simulink library "nmc"  (R2015b)
settings: Solver=ode45  SolverMode=SingleTasking  StartTime=0.0  StopTime=10.0  RelTol=1e-3
undefined symbols (not defined in the file): AFOFS_DIM, alphaFmGas, alphaFmGlu, alphaFmHam, alphaFmSol, alphaFmVas, alphaLceHam, alphaLceHfl, alphaLceTa, alphaLceTa1, Amp, amp_var, c, c_jointstop, CPG, D1G_HAT, DeltaThRef, eref, FmaxGAS, FmaxGLU, FmaxHAM, FmaxHFL, FmaxSOL, FmaxTA, FmaxVAS, freq, freq_var, GainDeltaTheta, GainGAS, GainGLU, GainHAM, GainHAMHFL, GainHFL, GainKneOverExt, GainSOL, GainSOLTA, GainTA, GainVAS, K, K_swing, KneePh23Offset, LceOffsetHAM, LceOffsetHFL, LceOffsetTA, left, LongDelay, loptGAS, loptGLU, loptHAM, loptHFL, loptSOL, loptTA, loptVAS, Lphi230, lslackGAS, lslackGLU, lslackHAM, lslackHFL, lslackSOL, lslackTA ... (+66)
libraries: nmc x94, simulink x29, simulink_extras x17
(part 3 of 5)

== system nmc/NMC Muscles/HFL&HAM Muscles/HFL&HAM Control ==
  note: HFL with HAM Control
  LceHFL : Inport
  LceHam : Inport  Port=2
  FmHam : Inport  Port=3
  Theta : Inport  Port=4
  dTheta : Inport  Port=5
  CLdxThigh : Inport  Port=6
  OLonCL : Inport  Port=7
  StanceSwing : Inport  Port=8
  "ANMC STIM " : Concatenate  NumInputs=1
  ANMC STIM 1 : Concatenate  NumInputs=1
  Demux : Demux  Outputs=2
  Logical Operator : Logic  Operator=NOT  AllPortsSameDT=off  OutDataTypeStr=boolean
  Mux1 : Mux  Inputs=2
  Mux2 : Mux  Inputs=2
  Saturation17 : Saturate  UpperLimit=1  LowerLimit=0.01  ZeroCross=off
  Stance Phase : Subsystem  TreatAsAtomicUnit=on
  Sum18 : Sum
  Swing Phase : Subsystem  TreatAsAtomicUnit=on
  StimHFL : Outport
  StimHAM : Outport  Port=2
  wires:
  ANMC STIM 1/1 -> StimHAM/1
  "ANMC STIM "/1 -> StimHFL/1
  Demux/1 -> "ANMC STIM "/1
  Demux/2 -> ANMC STIM 1/1
  OLonCL/1 -> Stance Phase/4(OLonCL)
  Swing Phase/2(StimHAM) -> Mux1/2
  Mux1/1 -> Sum18/2
  Mux2/1 -> Sum18/1
  Saturation17/1 -> Demux/1
  Sum18/1 -> Saturation17/1
  StanceSwing/1 -> Logical Operator/1, Stance Phase/Enable
  LceHFL/1 -> Swing Phase/2(LceHFL)
  Stance Phase/2(StimHAM) -> Mux2/2
  Stance Phase/1(StimHFL) -> Mux2/1
  CLdxThigh/1 -> Stance Phase/3(CLdxThigh [N])
  Stance Phase/3(Delta_Theta) -> Swing Phase/1(Delta_Theta)
  FmHam/1 -> Swing Phase/4(FmHAM)
  LceHam/1 -> Swing Phase/3(LceHAM)
  Swing Phase/1(StimHFL) -> Mux1/1
  dTheta/1 -> Stance Phase/2(dTheta [rad/s])
  Theta/1 -> Stance Phase/1(Theta)
  Logical Operator/1 -> Swing Phase/Enable

== system nmc/NMC Muscles/SOL&TA Muscles/SOL Actuation ==
  note: SOL Actuation
  phiAnkle : Inport
  StimSOL : Inport  Port=2
  " SOL" : Subsystem
  " SOL Golgi Tendon Organs" : Gain
  Mux3 : Mux  Inputs=5
  Product : Product  RndMeth=Zero
  SOL Link : Subsystem
  SOL loop delay : TransportDelay  DelayTime=LongDelay
  Terminator3 : Terminator
  TauSOL : Outport
  FmSOL : Outport  Port=2
  tag scope: SOLL_VM=global
  wires:
  SOL loop delay/1 -> FmSOL/1
  " SOL Golgi Tendon Organs"/1 -> SOL loop delay/1
  StimSOL/1 -> " SOL"/1(STIM)
  phiAnkle/1 -> SOL Link/1(phi12 [rad])
  " SOL"/4(Lse) -> Mux3/4
  " SOL"/3(Vce) -> Mux3/3
  " SOL"/2(Lce) -> Mux3/2
  Mux3/1 -> Terminator3/1, [SOLL_VM]
  " SOL"/5(A) -> Mux3/5
  Product/1 -> TauSOL/1
  SOL Link/2(lever [m]) -> Product/1
  SOL Link/1(lmtc [m]) -> " SOL"/2(lmtc [m])
  " SOL"/1(Fmtc) -> Mux3/1, " SOL Golgi Tendon Organs"/1, Product/2

== system nmc/NMC Muscles/SOL&TA Muscles/SOL&TA Control ==
  note: SOL with TA Control
  LceTA : Inport
  FmSOL : Inport  Port=2
  StanceSwing : Inport  Port=3
  " Stance Phase" : Subsystem  TreatAsAtomicUnit=on
  "ANMC STIM " : Concatenate  NumInputs=1
  ANMC STIM 1 : Concatenate  NumInputs=1
  Demux : Demux  Outputs=2
  Logical Operator : Logic  Operator=NOT  AllPortsSameDT=off  OutDataTypeStr=boolean
  Mux1 : Mux  Inputs=2
  Mux2 : Mux  Inputs=2
  Saturation17 : Saturate  UpperLimit=1  LowerLimit=0.01  ZeroCross=off
  Sum18 : Sum
  Swing Phase : Subsystem  TreatAsAtomicUnit=on
  StimTA : Outport
  StimSOL : Outport  Port=2
  wires:
  ANMC STIM 1/1 -> StimSOL/1
  "ANMC STIM "/1 -> StimTA/1
  Demux/1 -> "ANMC STIM "/1
  Demux/2 -> ANMC STIM 1/1
  Swing Phase/2(StimSOL) -> Mux1/2
  Mux1/1 -> Sum18/2
  Mux2/1 -> Sum18/1
  Saturation17/1 -> Demux/1
  Sum18/1 -> Saturation17/1
  " Stance Phase"/2(StimSOL) -> Mux2/2
  " Stance Phase"/1(StimTA) -> Mux2/1
  Swing Phase/1(StimTA) -> Mux1/1
  LceTA/1 -> " Stance Phase"/2(LceTA), Swing Phase/1(LceTA)
  StanceSwing/1 -> Logical Operator/1, " Stance Phase"/Enable
  FmSOL/1 -> " Stance Phase"/1(FmSOL)
  Logical Operator/1 -> Swing Phase/Enable

== system nmc/NMC Muscles/SOL&TA Muscles/TA Actuation ==
  note: TA Actuation
  phiAnkle : Inport
  StimTA : Inport  Port=2
  " TA Muscle Spindles" : Gain  Gain=1/loptTA
  " TA loop delay" : TransportDelay  DelayTime=LongDelay
  Gain : Gain  Gain=-1
  Mux8 : Mux  Inputs=5
  Product1 : Product  RndMeth=Zero
  Saturation2 : Saturate  UpperLimit=inf  LowerLimit=0  ZeroCross=off
  Stimulation Bias3 : Constant  Value=LceOffsetTA
  Sum21 : Sum  Inputs=-+|  SaturateOnIntegerOverflow=on  InputSameDT=on  OutDataTypeStr=Inherit: Same as first input
  TA : Subsystem
  TA Link : Subsystem
  Terminator8 : Terminator
  LceTA : Outport
  TauTa : Outport  Port=2
  tag scope: TAL_VM=global
  wires:
  Gain/1 -> TauTa/1
  " TA loop delay"/1 -> LceTA/1
  StimTA/1 -> TA/1(STIM)
  Product1/1 -> Gain/1
  Saturation2/1 -> " TA loop delay"/1
  Stimulation Bias3/1 -> Sum21/1
  phiAnkle/1 -> TA Link/1(phi12 [rad])
  TA/3(Vce) -> Mux8/3
  TA/4(Lse) -> Mux8/4
  Mux8/1 -> Terminator8/1, [TAL_VM]
  Sum21/1 -> Saturation2/1
  " TA Muscle Spindles"/1 -> Sum21/2
  TA Link/2(lever [m]) -> Product1/2
  TA Link/1(lmtc [m]) -> TA/2(lmtc [m])
  TA/5(A) -> Mux8/5
  TA/2(Lce) -> Mux8/2, " TA Muscle Spindles"/1
  TA/1(Fmtc) -> Mux8/1, Product1/1

== system nmc/NMC Muscles/VAS Muscle/VAS Actuation  ==
  note: VAS Actuation
  phiKnee : Inport
  StimVas : Inport  Port=2
  " VAS Golgi Tendon Organs" : Gain
  Gain : Gain  Gain=-1
  Mux9 : Mux  Inputs=5
  Product4 : Product  RndMeth=Zero
  Terminator9 : Terminator
  VAS : Subsystem
  VAS Link : Subsystem
  VAS loop delay : TransportDelay  DelayTime=MidDelay
  TauVas : Outport
  FmVas : Outport  Port=2
  tag scope: VASR_VM=global
  wires:
  VAS loop delay/1 -> FmVas/1
  " VAS Golgi Tendon Organs"/1 -> VAS loop delay/1
  Gain/1 -> TauVas/1
  StimVas/1 -> VAS/1(STIM)
  phiKnee/1 -> VAS Link/1(phi23 [rad])
  VAS/2(Lce) -> Mux9/2
  VAS/3(Vce) -> Mux9/3
  VAS/4(Lse) -> Mux9/4
  Mux9/1 -> Terminator9/1, [VASR_VM]
  VAS Link/2(lever [m]) -> Product4/1
  VAS/1(Fmtc) -> Mux9/1, " VAS Golgi Tendon Organs"/1, Product4/2
  VAS/5(A) -> Mux9/5
  Product4/1 -> Gain/1
  VAS Link/1(lmtu [m]) -> VAS/2(lmtc [m])

== system nmc/NMC Muscles/VAS Muscle/VAS Control ==
  note: VAS Control
  FmVAS : Inport
  OLdxThigh : Inport  Port=2
  OLonCL : Inport  Port=3
  CLKneeState : Inport  Port=4
  StanceSwing : Inport  Port=5
  " Swing Phase" : Subsystem  TreatAsAtomicUnit=on
  "ANMC STIM " : Concatenate  NumInputs=1
  Logical Operator : Logic  Operator=NOT  AllPortsSameDT=off  OutDataTypeStr=boolean
  Saturation17 : Saturate  UpperLimit=1  LowerLimit=0.01  ZeroCross=off
  Stance Phase : Subsystem  TreatAsAtomicUnit=on
  Sum18 : Sum
  StimVAS : Outport
  wires:
  "ANMC STIM "/1 -> StimVAS/1
  CLKneeState/1 -> Stance Phase/1(CLKneeState)
  OLonCL/1 -> Stance Phase/2(OLonCL)
  OLdxThigh/1 -> Stance Phase/3(OLdxThigh [N])
  Stance Phase/1(StimVAS) -> Sum18/1
  Saturation17/1 -> "ANMC STIM "/1
  Sum18/1 -> Saturation17/1
  " Swing Phase"/1(StimVAS) -> Sum18/2
  StanceSwing/1 -> Stance Phase/Enable, Logical Operator/1
  FmVAS/1 -> Stance Phase/4(FmVAS)
  Logical Operator/1 -> " Swing Phase"/Enable

== system nmc/NMC Sensors/FootSensor/Cross Influence Detection ==
  note: left leg is leading
  note: right leg is leading
  note: Double Support Cross Influences
  LStance : Inport  OutDataTypeStr=double
  RStance : Inport  Port=2  OutDataTypeStr=double
  DSup ends : HitCross  HitCrossingOffset=0.5  HitCrossingDirection=falling  ZeroCross=off
  Double Support? : Logic  AllPortsSameDT=off
  Double Support?1 : Logic  AllPortsSameDT=off
  Double Support?4 : Logic  AllPortsSameDT=off
  Flight? : Logic  Operator=NOR  AllPortsSameDT=off
  LLeg starts DSup : HitCross  HitCrossingOffset=0.5  HitCrossingDirection=rising  ZeroCross=off
  Memory : Memory
  Memory3 : Memory
  RLeg starts DSup : HitCross  HitCrossingOffset=0.5  HitCrossingDirection=rising  ZeroCross=off
  S-R Flip-Flop : simulink_extras/Flip Flops/S-R Flip-Flop  initial_condition=0
  S-R Flip-Flop1 : simulink_extras/Flip Flops/S-R Flip-Flop  initial_condition=0
  Terminator1 : Terminator
  Terminator2 : Terminator
  RonL : Outport  OutDataTypeStr=double
  Flight : Outport  Port=2  OutDataTypeStr=double
  LonR : Outport  Port=3  OutDataTypeStr=double
  wires:
  S-R Flip-Flop1/1 -> RonL/1
  Flight?/1 -> Flight/1
  S-R Flip-Flop/1 -> LonR/1
  Double Support?/1 -> Double Support?4/2, Double Support?1/1, DSup ends/1
  RStance/1 -> Flight?/2, Double Support?/2, Memory/1
  Memory3/1 -> LLeg starts DSup/1
  Double Support?4/1 -> S-R Flip-Flop/1
  LLeg starts DSup/1 -> Double Support?4/1
  LStance/1 -> Flight?/1, Double Support?/1, Memory3/1
  Memory/1 -> RLeg starts DSup/1
  S-R Flip-Flop1/2 -> Terminator2/1
  DSup ends/1 -> S-R Flip-Flop1/2, S-R Flip-Flop/2
  S-R Flip-Flop/2 -> Terminator1/1
  RLeg starts DSup/1 -> Double Support?1/2
  Double Support?1/1 -> S-R Flip-Flop1/1

== system nmc/NMC Sensors/FootSensor/Cross Influence Detection1 ==
  note: Double Support Cross Influences
  note: right leg is leading
  note: left leg is leading
  LStance : Inport  OutDataTypeStr=double
  RStance : Inport  Port=2  OutDataTypeStr=double
  Data Type Conversion{1..4} (4 alike) : DataTypeConversion
  Detect Decrease : simulink/Logic and Bit Operations/Detect Decrease  vinit=1.0  InputProcessing=Inherited  OutDataTypeStr=boolean
  Detect Increase : simulink/Logic and Bit Operations/Detect Increase  vinit=0.0  InputProcessing=Inherited  OutDataTypeStr=boolean
  Detect Increase1 : simulink/Logic and Bit Operations/Detect Increase  vinit=0.0  InputProcessing=Inherited  OutDataTypeStr=boolean
  Double Support? : Logic  AllPortsSameDT=off
  Double Support?1 : Logic  AllPortsSameDT=off
  Double Support?4 : Logic  AllPortsSameDT=off
  Flight? : Logic  Operator=NOR  AllPortsSameDT=off
  Memory : Memory
  Memory3 : Memory
  S-R Flip-Flop : simulink_extras/Flip Flops/S-R Flip-Flop  initial_condition=0
  S-R Flip-Flop1 : simulink_extras/Flip Flops/S-R Flip-Flop  initial_condition=0
  Terminator1 : Terminator
  Terminator2 : Terminator
  RonL : Outport  OutDataTypeStr=double
  Flight : Outport  Port=2  OutDataTypeStr=double
  LonR : Outport  Port=3  OutDataTypeStr=double
  wires:
  Double Support?1/1 -> S-R Flip-Flop1/1
  Detect Increase/1 -> Double Support?1/2
  S-R Flip-Flop/2 -> Terminator1/1
  S-R Flip-Flop1/2 -> Terminator2/1
  Memory/1 -> Detect Increase/1
  LStance/1 -> Memory3/1, Double Support?/1, Flight?/1
  Detect Increase1/1 -> Double Support?4/1
  Double Support?4/1 -> S-R Flip-Flop/1
  Memory3/1 -> Detect Increase1/1
  RStance/1 -> Memory/1, Double Support?/2, Flight?/2
  Double Support?/1 -> Data Type Conversion4/1, Double Support?1/1, Double Support?4/2
  S-R Flip-Flop/1 -> Data Type Conversion2/1
  Flight?/1 -> Data Type Conversion1/1
  S-R Flip-Flop1/1 -> Data Type Conversion3/1
  Data Type Conversion1/1 -> Flight/1
  Data Type Conversion2/1 -> LonR/1
  Data Type Conversion3/1 -> RonL/1
  Detect Decrease/1 -> S-R Flip-Flop/2, S-R Flip-Flop1/2
  Data Type Conversion4/1 -> Detect Decrease/1

== system nmc/Parameter variation/Alpha variation/Alpha Variation ==
  alpha : EnablePort  ShowOutputPort=on
  Gain : Gain  Gain=10
  Gain1 : Gain  Gain=0.1
  Ramp : simulink/Sources/Ramp  slope=0.05  start=2  X0=0
  Rounding Function : Rounding  Operator=round
  Saturation : Saturate  UpperLimit=1  LowerLimit=0
  Switch : Switch  Threshold=1
  "alphaOut " : Outport
  wires:
  Switch/1 -> "alphaOut "/1
  Ramp/1 -> Gain/1
  alpha/1 -> Switch/2, Switch/3
  Saturation/1 -> Switch/1
  Gain/1 -> Rounding Function/1
  Rounding Function/1 -> Gain1/1
  Gain1/1 -> Saturation/1

== system nmc/Parameter variation/Alpha variation/Alpha Variation1 ==
  alpha : EnablePort  ShowOutputPort=on
  Gain : Gain  Gain=10
  Gain1 : Gain  Gain=0.1
  Ramp : simulink/Sources/Ramp  slope=0.05  start=2  X0=0
  Rounding Function : Rounding  Operator=round
  Saturation : Saturate  UpperLimit=1  LowerLimit=0
  Switch : Switch  Threshold=1
  "alphaOut " : Outport
  wires:
  Switch/1 -> "alphaOut "/1
  Ramp/1 -> Gain/1
  alpha/1 -> Switch/2, Switch/3
  Saturation/1 -> Switch/1
  Gain/1 -> Rounding Function/1
  Rounding Function/1 -> Gain1/1
  Gain1/1 -> Saturation/1

== system nmc/Parameter variation/Alpha variation/Alpha Variation2 ==
  alpha : EnablePort  ShowOutputPort=on
  Gain : Gain  Gain=10
  Gain1 : Gain  Gain=0.1
  Ramp : simulink/Sources/Ramp  slope=0.05  start=2  X0=0
  Rounding Function : Rounding  Operator=round
  Saturation : Saturate  UpperLimit=1  LowerLimit=0
  Switch : Switch  Threshold=1
  "alphaOut " : Outport
  wires:
  Switch/1 -> "alphaOut "/1
  Ramp/1 -> Gain/1
  alpha/1 -> Switch/2, Switch/3
  Saturation/1 -> Switch/1
  Gain/1 -> Rounding Function/1
  Rounding Function/1 -> Gain1/1
  Gain1/1 -> Saturation/1

== system nmc/Parameter variation/Alpha variation/Alpha Variation3 ==
  alpha : EnablePort  ShowOutputPort=on
  Gain : Gain  Gain=10
  Gain1 : Gain  Gain=0.1
  Ramp : simulink/Sources/Ramp  slope=0.05  start=2  X0=0
  Rounding Function : Rounding  Operator=round
  Saturation : Saturate  UpperLimit=1  LowerLimit=0
  Switch : Switch  Threshold=1
  "alphaOut " : Outport
  wires:
  Switch/1 -> "alphaOut "/1
  Ramp/1 -> Gain/1
  alpha/1 -> Switch/2, Switch/3
  Saturation/1 -> Switch/1
  Gain/1 -> Rounding Function/1
  Rounding Function/1 -> Gain1/1
  Gain1/1 -> Saturation/1

== system nmc/Parameter variation/Alpha variation/Alpha Variation4 ==
  alpha : EnablePort  ShowOutputPort=on
  Gain : Gain  Gain=10
  Gain1 : Gain  Gain=0.1
  Ramp : simulink/Sources/Ramp  slope=0.05  start=2  X0=0
  Rounding Function : Rounding  Operator=round
  Saturation : Saturate  UpperLimit=1  LowerLimit=0
  Switch : Switch  Threshold=1
  "alphaOut " : Outport
  wires:
  Switch/1 -> "alphaOut "/1
  Ramp/1 -> Gain/1
  alpha/1 -> Switch/2, Switch/3
  Saturation/1 -> Switch/1
  Gain/1 -> Rounding Function/1
  Rounding Function/1 -> Gain1/1
  Gain1/1 -> Saturation/1

== system nmc/Parameter variation/Alpha variation/Alpha Variation5 ==
  alpha : EnablePort  ShowOutputPort=on
  Gain : Gain  Gain=10
  Gain1 : Gain  Gain=0.1
  Ramp : simulink/Sources/Ramp  slope=0.05  start=2  X0=0
  Rounding Function : Rounding  Operator=round
  Saturation : Saturate  UpperLimit=1  LowerLimit=0
  Switch : Switch  Threshold=1
  "alphaOut " : Outport
  wires:
  Switch/1 -> "alphaOut "/1
  Ramp/1 -> Gain/1
  alpha/1 -> Switch/2, Switch/3
  Saturation/1 -> Switch/1
  Gain/1 -> Rounding Function/1
  Rounding Function/1 -> Gain1/1
  Gain1/1 -> Saturation/1

== system nmc/Parameter variation/Alpha variation/Alpha Variation6 ==
  alpha : EnablePort  ShowOutputPort=on
  Gain : Gain  Gain=10
  Gain1 : Gain  Gain=0.1
  Ramp : simulink/Sources/Ramp  slope=0.05  start=2  X0=0
  Rounding Function : Rounding  Operator=round
  Saturation : Saturate  UpperLimit=1  LowerLimit=0
  Switch : Switch  Threshold=1
  "alphaOut " : Outport
  wires:
  Switch/1 -> "alphaOut "/1
  Ramp/1 -> Gain/1
  alpha/1 -> Switch/2, Switch/3
  Saturation/1 -> Switch/1
  Gain/1 -> Rounding Function/1
  Rounding Function/1 -> Gain1/1
  Gain1/1 -> Saturation/1

== system nmc/Parameter variation/Alpha variation/Alpha Variation7 ==
  alpha : EnablePort  ShowOutputPort=on
  Gain : Gain  Gain=10
  Gain1 : Gain  Gain=0.1
  Ramp : simulink/Sources/Ramp  slope=0.05  start=2  X0=0
  Rounding Function : Rounding  Operator=round
  Saturation : Saturate  UpperLimit=1  LowerLimit=0
  Switch : Switch  Threshold=1
  "alphaOut " : Outport
  wires:
  Switch/1 -> "alphaOut "/1
  Ramp/1 -> Gain/1
  alpha/1 -> Switch/2, Switch/3
  Saturation/1 -> Switch/1
  Gain/1 -> Rounding Function/1
  Rounding Function/1 -> Gain1/1
  Gain1/1 -> Saturation/1

== system nmc/Parameter variation/Alpha variation/Alpha Variation8 ==
  alpha : EnablePort  ShowOutputPort=on
  Gain : Gain  Gain=10
  Gain1 : Gain  Gain=0.1
  Ramp : simulink/Sources/Ramp  slope=0.05  start=2  X0=0
  Rounding Function : Rounding  Operator=round
  Saturation : Saturate  UpperLimit=1  LowerLimit=0
  Switch : Switch  Threshold=1
  "alphaOut " : Outport
  wires:
  Switch/1 -> "alphaOut "/1
  Ramp/1 -> Gain/1
  alpha/1 -> Switch/2, Switch/3
  Saturation/1 -> Switch/1
  Gain/1 -> Rounding Function/1
  Rounding Function/1 -> Gain1/1
  Gain1/1 -> Saturation/1

== system nmc/Parameter variation/Amplitude Variation/Down ==
  Amp : Inport
  Enable : EnablePort
  Gain : Gain  Gain=10
  Gain1 : Gain  Gain=0.1
  Ramp : simulink/Sources/Ramp  slope=0.04  start=2  X0=0
  Rounding Function : Rounding  Operator=round
  Saturation : Saturate  UpperLimit=1.5  LowerLimit=0
  Subtract : Sum  Inputs=+-
  "AmpDown " : Outport
  wires:
  Saturation/1 -> Subtract/2
  Ramp/1 -> Gain/1
  Amp/1 -> Subtract/1
  Gain/1 -> Rounding Function/1
  Rounding Function/1 -> Gain1/1
  Gain1/1 -> Saturation/1
  Subtract/1 -> "AmpDown "/1

== system nmc/Parameter variation/Amplitude Variation/Off  ==
  Amp : Inport
  Enable : EnablePort
  "Amp " : Outport
  wires:
  Amp/1 -> "Amp "/1

== system nmc/Parameter variation/Amplitude Variation/Up ==
  Amp : Inport
  Enable : EnablePort
  Gain : Gain  Gain=10
  Gain1 : Gain  Gain=0.1
  Ramp : simulink/Sources/Ramp  slope=0.04  start=2  X0=0
  Rounding Function : Rounding  Operator=round
  Saturation : Saturate  UpperLimit=1.5  LowerLimit=0
  Sum : Sum  Inputs=|++
  "AmpUp " : Outport
  wires:
  Ramp/1 -> Gain/1
  Gain/1 -> Rounding Function/1
  Rounding Function/1 -> Gain1/1
  Gain1/1 -> Saturation/1
  Sum/1 -> "AmpUp "/1
  Saturation/1 -> Sum/1
  Amp/1 -> Sum/2

== system nmc/Parameter variation/Freq variation/Down ==
  "freq " : Inport
  Enable : EnablePort
  Gain : Gain  Gain=10
  Gain1 : Gain  Gain=0.1
  Ramp : simulink/Sources/Ramp  slope=0.04  start=2  X0=0
  Rounding Function : Rounding  Operator=round
  Saturation : Saturate  UpperLimit=1.5  LowerLimit=0
  Subtract : Sum  Inputs=+-
  "freqDown " : Outport
  wires:
  Saturation/1 -> Subtract/2
  Ramp/1 -> Gain/1
  "freq "/1 -> Subtract/1
  Gain/1 -> Rounding Function/1
  Rounding Function/1 -> Gain1/1
  Gain1/1 -> Saturation/1
  Subtract/1 -> "freqDown "/1

== system nmc/Parameter variation/Freq variation/Off  ==
  freq : Inport
  Enable : EnablePort
  "Amp " : Outport
  wires:
  freq/1 -> "Amp "/1

== system nmc/Parameter variation/Freq variation/Up ==
  "freq " : Inport
  Enable : EnablePort
  Gain : Gain  Gain=10
  Gain1 : Gain  Gain=0.1
  Ramp : simulink/Sources/Ramp  slope=0.04  start=2  X0=0
  Rounding Function : Rounding  Operator=round
  Saturation : Saturate  UpperLimit=1.5  LowerLimit=0
  Sum : Sum  Inputs=|++
  "freqUp " : Outport
  wires:
  Ramp/1 -> Gain/1
  Gain/1 -> Rounding Function/1
  Rounding Function/1 -> Gain1/1
  Gain1/1 -> Saturation/1
  Sum/1 -> "freqUp "/1
  Saturation/1 -> Sum/1
  "freq "/1 -> Sum/2

== system nmc/VAS Muscle/VAS Actuation /VAS ==
  note: VASTI Muscle-Tendon Dynamics
  note: Excitation Contraction Coupling
  STIM : Inport
  lmtc [m] : Inport  Port=2
  1 : Product  Inputs=**  SaturateOnIntegerOverflow=on  InputSameDT=on  OutDataTypeStr=Inherit: Same as first input
  1/lslack : Gain  Gain=1/lslackVAS  SaturateOnIntegerOverflow=on  OutDataTypeStr=Inherit: Same as input  ParamDataTypeStr=Inherit: Same as input
  BE force-length relation : Subsystem
  CE force-length relation : Subsystem
  CE inverse force-velocity relation : Subsystem
  Constant : Constant  Value=lslackVAS
  ECC TransferFcn : simulink_extras/Additional Linear/Transfer Fcn (with initial outputs)  N=[1]  D="[tau  1]"  Y0=preA  U0=0
      settings: AttributesFormatString=pre-activation: %<Y0>
  Fmax : Gain  Gain=FmaxVAS  SaturateOnIntegerOverflow=on  OutDataTypeStr=Inherit: Same as input  ParamDataTypeStr=Inherit: Same as input
  Fv = Fse / (A*Fce) : Product  Inputs=*/  SaturateOnIntegerOverflow=on  InputSameDT=on  OutDataTypeStr=Inherit: Same as first input
  Integrator : Integrator  InitialConditionSource=external  LowerSaturationLimit=0.05
  PE force-length relation : Subsystem
  SE force-length relation : Subsystem
  Sum : Sum  Inputs=|+-  SaturateOnIntegerOverflow=on  InputSameDT=on  OutDataTypeStr=Inherit: Same as first input
  Sum2 : Sum  Inputs=|-+  SaturateOnIntegerOverflow=on  InputSameDT=on  OutDataTypeStr=Inherit: Same as first input
  Sum3 : Sum  SaturateOnIntegerOverflow=on  InputSameDT=on  OutDataTypeStr=Inherit: Same as first input
  Sum4 : Sum  SaturateOnIntegerOverflow=on  InputSameDT=on  OutDataTypeStr=Inherit: Same as first input
  lce/lopt : Gain  Gain=1/loptVAS  SaturateOnIntegerOverflow=on  OutDataTypeStr=Inherit: Same as input  ParamDataTypeStr=Inherit: Same as input
  vmax*lopt : Gain  Gain=vmaxVAS*loptVAS  SaturateOnIntegerOverflow=on  OutDataTypeStr=Inherit: Same as input  ParamDataTypeStr=Inherit: Same as input
  Fmtc : Outport  InitialOutput=0
  Lce : Outport  Port=2  InitialOutput=0
  Vce : Outport  Port=3  InitialOutput=0
  Lse : Outport  Port=4  InitialOutput=0
  A : Outport  Port=5  InitialOutput=0
  wires:
  Integrator/1 -> Sum/2, lce/lopt/1, Lce/1  "lce"
  Sum/1 -> 1/lslack/1, Lse/1  "lse"
  lce/lopt/1 -> CE force-length relation/1(lce [lopt]), BE force-length relation/1(lce [lopt]), PE force-length relation/1(lce [lopt])
  Fv = Fse / (A*Fce)/1 -> CE inverse force-velocity relation/1(Fv[Fmax])  "fv"
  vmax*lopt/1 -> Integrator/1, Vce/1  "vce"
  lmtc [m]/1 -> Sum2/2, Sum/1  "lmtc"
  Fmax/1 -> Fmtc/1  "Fmtc"
  1/lslack/1 -> SE force-length relation/1(lse [lslack])
  SE force-length relation/1(fse [Fmax]) -> Fmax/1, Sum4/1
  Sum2/1 -> Integrator/2
  Constant/1 -> Sum2/1
  CE force-length relation/1(fce [Fmax]) -> 1/1
  Sum4/1 -> Fv = Fse / (A*Fce)/1
  PE force-length relation/1(fpe [Fmax]) -> Sum3/1
  1/1 -> Sum3/2
  BE force-length relation/1(fbe [Fmax]) -> Sum4/2
  Sum3/1 -> Fv = Fse / (A*Fce)/2
  CE inverse force-velocity relation/1(v[vmax]) -> vmax*lopt/1
  STIM/1 -> ECC TransferFcn/1
  ECC TransferFcn/1 -> 1/2, A/1

== system nmc/VAS Muscle/VAS Actuation /VAS Link ==
  note: Muscle Length and Moment Arm
  phi23 [rad] : Inport
  Constant : Constant  Value=lslackVAS+loptVAS
  Constant2 : Constant  Value=phirefVAS
  Constant3 : Constant  Value=phimaxVAS
  Demux : Demux  Outputs=2
  Gain2 : Gain  Gain=rVAS
  Gain4 : Gain  Gain=rhoVAS
  Mux : Mux  Inputs=2
  Sum2 : Sum  Inputs=|+-
  Sum3 : Sum  Inputs=-+|
  Sum4 : Sum  Inputs=+-
  Sum5 : Sum  Inputs=|++
  length change term : Trigonometry
  offset correction term : Trigonometry
  variable lever term : Trigonometry  Operator=cos
  lmtu [m] : Outport
  lever [m] : Outport  Port=2
  wires:
  phi23 [rad]/1 -> Sum3/2
  Sum3/1 -> variable lever term/1, length change term/1
  Constant3/1 -> Sum3/1, Sum2/2
  Sum2/1 -> offset correction term/1
  Constant2/1 -> Sum2/1
  length change term/1 -> Sum4/2
  offset correction term/1 -> Sum4/1
  Sum4/1 -> Mux/1
  Constant/1 -> Sum5/1
  Sum5/1 -> lmtu [m]/1
  Gain4/1 -> Sum5/2
  variable lever term/1 -> Mux/2
  Mux/1 -> Gain2/1
  Gain2/1 -> Demux/1
  Demux/1 -> Gain4/1
  Demux/2 -> lever [m]/1

== system nmc/Full Body Control/Left Side/AnkleJoint left/ Ankle Joint Limits ==
  note: Ankle Joint Limits
  phi [rad] : Inport
  dphi [rad/s] : Inport  Port=2
  Gain1 : Gain  Gain=c_jointstop
  Gain2 : Gain  Gain=-1
  Gain3 : Gain  Gain=c_jointstop
  Gain4 : Gain  Gain=1/w_max_jointstop
  Limit Ankle Range : simulink/Logic and Bit Operations/Interval Test  IntervalClosedRight=on  uplimit=phi12_UpLimit + 40*pi/180  IntervalClosedLeft=on  lowlimit=phi12_LowLimit - 40*pi/180  OutDataTypeStr=boolean
  Logical Operator3 : Logic  Operator=NOT  AllPortsSameDT=off  OutDataTypeStr=boolean
  Mux1 : Mux  Inputs=2
  Mux3 : Mux  Inputs=2
  Overextension Torque : Fcn  Expr="- u(1)  *  (1-u(2)) * (u(2)<1) * (u(1)>0)"
  Overflexion Torque : Fcn  Expr="- u(1)  *  (1-u(2)) * (u(2)<1) * (u(1)<0)"
  Stop Simulation1 : Stop
  Sum : Sum  Inputs=|+-
  Sum1 : Sum  Inputs=|+-
  Sum2 : Sum
  overextension angle : Constant  Value=phi12_UpLimit
  overflexion angle : Constant  Value=phi12_LowLimit
  M_stop [Nm] : Outport
  wires:
  Logical Operator3/1 -> Stop Simulation1/1
  Limit Ankle Range/1 -> Logical Operator3/1
  Overextension Torque/1 -> Sum2/1
  Overflexion Torque/1 -> Sum2/2
  Gain2/1 -> Mux3/2
  Sum2/1 -> M_stop [Nm]/1
  Mux1/1 -> Overflexion Torque/1
  overflexion angle/1 -> Sum1/2
  Sum1/1 -> Gain1/1
  Gain1/1 -> Mux1/1
  Gain4/1 -> Mux1/2, Gain2/1
  Sum/1 -> Gain3/1
  phi [rad]/1 -> Limit Ankle Range/1, Sum1/1, Sum/1
  overextension angle/1 -> Sum/2
  dphi [rad/s]/1 -> Gain4/1
  Gain3/1 -> Mux3/1
  Mux3/1 -> Overextension Torque/1

== system nmc/Full Body Control/Left Side/HipJoint left/Hip Joint Limits ==
  note: Hip Joint Limits
  phi [rad] : Inport
  dphi [rad/s] : Inport  Port=2
  Gain2 : Gain  Gain=-1
  Gain3 : Gain  Gain=c_jointstop
  Gain4 : Gain  Gain=1/w_max_jointstop
  Limit Hip Range : simulink/Logic and Bit Operations/Interval Test  IntervalClosedRight=on  uplimit=phi34_UpLimit + 30*pi/180  IntervalClosedLeft=on  lowlimit=10*pi/180  OutDataTypeStr=boolean
  Logical Operator3 : Logic  Operator=NOT  AllPortsSameDT=off  OutDataTypeStr=boolean
  Mux3 : Mux  Inputs=2
  Overextension Torque : Fcn  Expr="- u(1)  *  (1-u(2)) * (u(2)<1) * (u(1)>0)"
  Stop Simulation1 : Stop
  Sum : Sum  Inputs=|+-
  overextension angle : Constant  Value=phi34_UpLimit
  M_stop [Nm] : Outport
  wires:
  Logical Operator3/1 -> Stop Simulation1/1
  Limit Hip Range/1 -> Logical Operator3/1
  Overextension Torque/1 -> M_stop [Nm]/1
  Gain2/1 -> Mux3/2
  Gain4/1 -> Gain2/1
  Sum/1 -> Gain3/1
  phi [rad]/1 -> Limit Hip Range/1, Sum/1
  overextension angle/1 -> Sum/2
  dphi [rad/s]/1 -> Gain4/1
  Gain3/1 -> Mux3/1
  Mux3/1 -> Overextension Torque/1

== system nmc/Full Body Control/Left Side/KneeJoint left/Knee Joint Limits ==
  note: Knee Joint Limits
  phi [rad] : Inport
  dphi [rad/s] : Inport  Port=2
  Gain2 : Gain  Gain=-1
  Gain3 : Gain  Gain=c_jointstop
  Gain4 : Gain  Gain=1/w_max_jointstop
  Limit Knee Range : simulink/Logic and Bit Operations/Interval Test  IntervalClosedRight=on  uplimit=185*pi/180  IntervalClosedLeft=on  lowlimit=40*pi/180  OutDataTypeStr=boolean
  Logical Operator3 : Logic  Operator=NOT  AllPortsSameDT=off  OutDataTypeStr=boolean
  Mux3 : Mux  Inputs=2
  Overextension Torque : Fcn  Expr="- u(1)  *  (1-u(2)) * (u(2)<1) * (u(1)>0)"
  Stop Simulation1 : Stop
  Sum : Sum  Inputs=|+-
  overextension angle : Constant  Value=phi23_UpLimit
  M_stop [Nm] : Outport
  wires:
  Logical Operator3/1 -> Stop Simulation1/1
  Limit Knee Range/1 -> Logical Operator3/1
  Overextension Torque/1 -> M_stop [Nm]/1
  Gain2/1 -> Mux3/2
  Gain4/1 -> Gain2/1
  Sum/1 -> Gain3/1
  phi [rad]/1 -> Limit Knee Range/1, Sum/1
  overextension angle/1 -> Sum/2
  dphi [rad/s]/1 -> Gain4/1
  Gain3/1 -> Mux3/1
  Mux3/1 -> Overextension Torque/1

== system nmc/Lopes/Left Side/HipJoint left/Hip Joint Limits ==
  note: Hip Joint Limits
  phi [rad] : Inport
  dphi [rad/s] : Inport  Port=2
  Gain2 : Gain  Gain=-1
  Gain3 : Gain  Gain=c_jointstop
  Gain4 : Gain  Gain=1/w_max_jointstop
  Limit Hip Range : simulink/Logic and Bit Operations/Interval Test  IntervalClosedRight=on  uplimit=phi34_UpLimit + 30*pi/180  IntervalClosedLeft=on  lowlimit=10*pi/180  OutDataTypeStr=boolean
  Logical Operator3 : Logic  Operator=NOT  AllPortsSameDT=off  OutDataTypeStr=boolean
  Mux3 : Mux  Inputs=2
  Overextension Torque : Fcn  Expr="- u(1)  *  (1-u(2)) * (u(2)<1) * (u(1)>0)"
  Stop Simulation1 : Stop
  Sum : Sum  Inputs=|+-
  overextension angle : Constant  Value=phi34_UpLimit
  M_stop [Nm] : Outport
  wires:
  Logical Operator3/1 -> Stop Simulation1/1
  Limit Hip Range/1 -> Logical Operator3/1
  Overextension Torque/1 -> M_stop [Nm]/1
  Gain2/1 -> Mux3/2
  Gain4/1 -> Gain2/1
  Sum/1 -> Gain3/1
  phi [rad]/1 -> Limit Hip Range/1, Sum/1
  overextension angle/1 -> Sum/2
  dphi [rad/s]/1 -> Gain4/1
  Gain3/1 -> Mux3/1
  Mux3/1 -> Overextension Torque/1

== system nmc/Lopes/Left Side/KneeJoint left/Knee Joint Limits ==
  note: Knee Joint Limits
  phi [rad] : Inport
  dphi [rad/s] : Inport  Port=2
  Gain2 : Gain  Gain=-1
  Gain3 : Gain  Gain=c_jointstop
  Gain4 : Gain  Gain=1/w_max_jointstop
  Limit Knee Range : simulink/Logic and Bit Operations/Interval Test  IntervalClosedRight=on  uplimit=185*pi/180  IntervalClosedLeft=on  lowlimit=40*pi/180  OutDataTypeStr=boolean
  Logical Operator3 : Logic  Operator=NOT  AllPortsSameDT=off  OutDataTypeStr=boolean
  Mux3 : Mux  Inputs=2
  Overextension Torque : Fcn  Expr="- u(1)  *  (1-u(2)) * (u(2)<1) * (u(1)>0)"
  Stop Simulation1 : Stop
  Sum : Sum  Inputs=|+-
  overextension angle : Constant  Value=phi23_UpLimit
  M_stop [Nm] : Outport
  wires:
  Logical Operator3/1 -> Stop Simulation1/1
  Limit Knee Range/1 -> Logical Operator3/1
  Overextension Torque/1 -> M_stop [Nm]/1
  Gain2/1 -> Mux3/2
  Gain4/1 -> Gain2/1
  Sum/1 -> Gain3/1
  phi [rad]/1 -> Limit Knee Range/1, Sum/1
  overextension angle/1 -> Sum/2
  dphi [rad/s]/1 -> Gain4/1
  Gain3/1 -> Mux3/1
  Mux3/1 -> Overextension Torque/1

== system nmc/NMC Muscles/GAS Muscle/GAS Actuation / GAS ==
  note: Excitation Contraction Coupling
  note: SOLEUS Muscle-Tendon Dynamics
  STIM : Inport
  lmtc [m] : Inport  Port=2
  1 : Product  Inputs=**  SaturateOnIntegerOverflow=on  InputSameDT=on  OutDataTypeStr=Inherit: Same as first input
  1/lslack : Gain  Gain=1/lslackGAS  SaturateOnIntegerOverflow=on  OutDataTypeStr=Inherit: Same as input  ParamDataTypeStr=Inherit: Same as input
  BE force-length relation : Subsystem
  CE force-length relation : Subsystem
  CE inverse force-velocity relation : Subsystem
  Constant : Constant  Value=lslackGAS
  ECC TransferFcn : simulink_extras/Additional Linear/Transfer Fcn (with initial outputs)  N=[1]  D=[tau 1]  Y0=preA  U0=0
      settings: AttributesFormatString=pre-activation: %<Y0>
  Fmax : Gain  Gain=FmaxGAS  SaturateOnIntegerOverflow=on  OutDataTypeStr=Inherit: Same as input  ParamDataTypeStr=Inherit: Same as input
  Fv = Fse / (A*Fce) : Product  Inputs=*/  SaturateOnIntegerOverflow=on  InputSameDT=on  OutDataTypeStr=Inherit: Same as first input
  Integrator : Integrator  InitialConditionSource=external  LowerSaturationLimit=0.05
  PE force-length relation : Subsystem
  SE force-length relation : Subsystem
  Sum : Sum  Inputs=|+-  SaturateOnIntegerOverflow=on  InputSameDT=on  OutDataTypeStr=Inherit: Same as first input
  Sum2 : Sum  Inputs=|-+  SaturateOnIntegerOverflow=on  InputSameDT=on  OutDataTypeStr=Inherit: Same as first input
  Sum3 : Sum  SaturateOnIntegerOverflow=on  InputSameDT=on  OutDataTypeStr=Inherit: Same as first input
  Sum4 : Sum  SaturateOnIntegerOverflow=on  InputSameDT=on  OutDataTypeStr=Inherit: Same as first input
  lce/lopt : Gain  Gain=1/loptGAS  SaturateOnIntegerOverflow=on  OutDataTypeStr=Inherit: Same as input  ParamDataTypeStr=Inherit: Same as input
  vmax*lopt : Gain  Gain=vmaxGAS*loptGAS  SaturateOnIntegerOverflow=on  OutDataTypeStr=Inherit: Same as input  ParamDataTypeStr=Inherit: Same as input
  Fmtc : Outport  InitialOutput=0
  Lce : Outport  Port=2  InitialOutput=0
  Vce : Outport  Port=3  InitialOutput=0
  Lse : Outport  Port=4  InitialOutput=0
  A : Outport  Port=5  InitialOutput=0
  wires:
  ECC TransferFcn/1 -> 1/2, A/1
  STIM/1 -> ECC TransferFcn/1
  CE inverse force-velocity relation/1(v[vmax]) -> vmax*lopt/1
  Sum3/1 -> Fv = Fse / (A*Fce)/2
  BE force-length relation/1(fbe [Fmax]) -> Sum4/2
  1/1 -> Sum3/2
  PE force-length relation/1(fpe [Fmax]) -> Sum3/1
  Sum4/1 -> Fv = Fse / (A*Fce)/1
  CE force-length relation/1(fce [Fmax]) -> 1/1
  Constant/1 -> Sum2/1
  Sum2/1 -> Integrator/2
  SE force-length relation/1(fse [Fmax]) -> Sum4/1, Fmax/1
  1/lslack/1 -> SE force-length relation/1(lse [lslack])
  Fmax/1 -> Fmtc/1  "Fmtc"
  lmtc [m]/1 -> Sum/1, Sum2/2  "lmtc"
  vmax*lopt/1 -> Vce/1, Integrator/1  "vce"
  Fv = Fse / (A*Fce)/1 -> CE inverse force-velocity relation/1(Fv[Fmax])  "fv"
  lce/lopt/1 -> PE force-length relation/1(lce [lopt]), BE force-length relation/1(lce [lopt]), CE force-length relation/1(lce [lopt])
  Sum/1 -> Lse/1, 1/lslack/1  "lse"
  Integrator/1 -> Lce/1, lce/lopt/1, Sum/2  "lce"

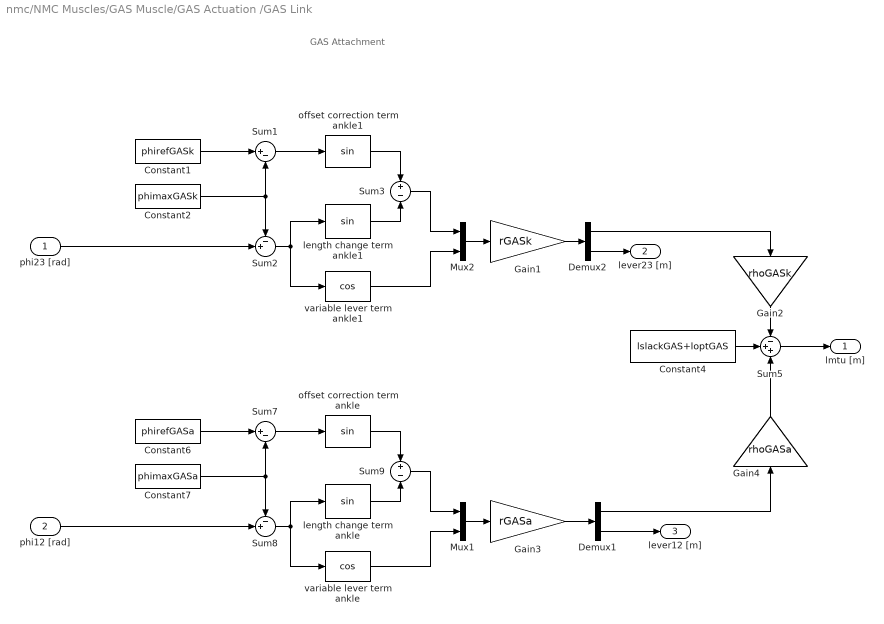
== system nmc/NMC Muscles/GAS Muscle/GAS Actuation /GAS Link ==
  note: GAS Attachment
  phi23 [rad] : Inport
  phi12 [rad] : Inport  Port=2
  Constant1 : Constant  Value=phirefGASk
  Constant2 : Constant  Value=phimaxGASk
  Constant4 : Constant  Value=lslackGAS+loptGAS
  Constant6 : Constant  Value=phirefGASa
  Constant7 : Constant  Value=phimaxGASa
  Demux1 : Demux  Outputs=2
  Demux2 : Demux  Outputs=2
  Gain1 : Gain  Gain=rGASk
  Gain2 : Gain  Gain=rhoGASk
  Gain3 : Gain  Gain=rGASa
  Gain4 : Gain  Gain=rhoGASa
  Mux1 : Mux  Inputs=2
  Mux2 : Mux  Inputs=2
  Sum1 : Sum  Inputs=|+-
  Sum2 : Sum  Inputs=-+|
  Sum3 : Sum  Inputs=+-
  Sum5 : Sum  Inputs=-++
  Sum7 : Sum  Inputs=|+-
  Sum8 : Sum  Inputs=-+|
  Sum9 : Sum  Inputs=+-
  length change term ankle : Trigonometry
  length change term ankle1 : Trigonometry
  offset correction term ankle : Trigonometry
  offset correction term ankle1 : Trigonometry
  variable lever term ankle : Trigonometry  Operator=cos
  variable lever term ankle1 : Trigonometry  Operator=cos
  lmtu [m] : Outport
  lever23 [m] : Outport  Port=2
  lever12 [m] : Outport  Port=3
  wires:
  Gain2/1 -> Sum5/1
  Demux2/1 -> Gain2/1
  Demux2/2 -> lever23 [m]/1
  Gain1/1 -> Demux2/1
  Mux2/1 -> Gain1/1
  Sum3/1 -> Mux2/1
  offset correction term ankle1/1 -> Sum3/1
  length change term ankle1/1 -> Sum3/2
  Constant1/1 -> Sum1/1
  Sum1/1 -> offset correction term ankle1/1
  Constant2/1 -> Sum1/2, Sum2/1
  Sum2/1 -> length change term ankle1/1, variable lever term ankle1/1
  variable lever term ankle1/1 -> Mux2/2
  phi23 [rad]/1 -> Sum2/2
  Gain4/1 -> Sum5/3
  Demux1/1 -> Gain4/1
  Gain3/1 -> Demux1/1
  Mux1/1 -> Gain3/1
  Constant4/1 -> Sum5/2
  Sum9/1 -> Mux1/1
  offset correction term ankle/1 -> Sum9/1
  length change term ankle/1 -> Sum9/2
  Constant6/1 -> Sum7/1
  Sum7/1 -> offset correction term ankle/1
  Constant7/1 -> Sum7/2, Sum8/1
  Sum8/1 -> length change term ankle/1, variable lever term ankle/1
  Demux1/2 -> lever12 [m]/1
  variable lever term ankle/1 -> Mux1/2
  Sum5/1 -> lmtu [m]/1
  phi12 [rad]/1 -> Sum8/2

== system nmc/NMC Muscles/GAS Muscle/GAS Control/ Swing Phase ==
  note: Swing Phase Control
  note: GAS Control
  Enable : EnablePort  StatesWhenEnabling=reset
  Stimulation Bias1 : Constant  Value=PreStimGAS
  StimGAS : Outport  OutputWhenDisabled=reset  InitialOutput=0
  wires:
  Stimulation Bias1/1 -> StimGAS/1

== system nmc/NMC Muscles/GAS Muscle/GAS Control/Stance Phase ==
  note: Stance Phase Control
  note: GAS Control
  FmGAS : Inport
  Enable : EnablePort  StatesWhenEnabling=reset
  FB Gain2 : Gain  Gain=GainGAS  SaturateOnIntegerOverflow=on  OutDataTypeStr=Inherit: Same as input  ParamDataTypeStr=Inherit: Same as input
  Stimulation Bias1 : Constant  Value=PreStimGAS
  Sum3 : Sum  Inputs=|++  SaturateOnIntegerOverflow=on  InputSameDT=on  OutDataTypeStr=Inherit: Same as first input
  StimGAS : Outport  OutputWhenDisabled=reset  InitialOutput=0
  wires:
  FB Gain2/1 -> Sum3/2
  Sum3/1 -> StimGAS/1
  Stimulation Bias1/1 -> Sum3/1
  FmGAS/1 -> FB Gain2/1

== system nmc/NMC Muscles/GLU Muscle/GLU Actuation/ GLU ==
  note: Excitation Contraction Coupling
  note: SOLEUS Muscle-Tendon Dynamics
  STIM : Inport
  lmtc [m] : Inport  Port=2
  1 : Product  Inputs=**  SaturateOnIntegerOverflow=on  InputSameDT=on  OutDataTypeStr=Inherit: Same as first input
  1/lslack : Gain  Gain=1/lslackGLU  SaturateOnIntegerOverflow=on  OutDataTypeStr=Inherit: Same as input  ParamDataTypeStr=Inherit: Same as input
  BE force-length relation : Subsystem
  CE force-length relation : Subsystem
  CE inverse force-velocity relation : Subsystem
  Constant : Constant  Value=lslackGLU
  ECC TransferFcn : simulink_extras/Additional Linear/Transfer Fcn (with initial outputs)  N=[1]  D="[tau  1]"  Y0=preA  U0=0
      settings: AttributesFormatString=pre-activation: %<Y0>
  Fmax : Gain  Gain=FmaxGLU  SaturateOnIntegerOverflow=on  OutDataTypeStr=Inherit: Same as input  ParamDataTypeStr=Inherit: Same as input
  Fv = Fse / (A*Fce) : Product  Inputs=*/  SaturateOnIntegerOverflow=on  InputSameDT=on  OutDataTypeStr=Inherit: Same as first input
  Integrator : Integrator  InitialConditionSource=external  LowerSaturationLimit=0.05
  PE force-length relation : Subsystem
  SE force-length relation : Subsystem
  Sum : Sum  Inputs=|+-  SaturateOnIntegerOverflow=on  InputSameDT=on  OutDataTypeStr=Inherit: Same as first input
  Sum2 : Sum  Inputs=|-+  SaturateOnIntegerOverflow=on  InputSameDT=on  OutDataTypeStr=Inherit: Same as first input
  Sum3 : Sum  SaturateOnIntegerOverflow=on  InputSameDT=on  OutDataTypeStr=Inherit: Same as first input
  Sum4 : Sum  SaturateOnIntegerOverflow=on  InputSameDT=on  OutDataTypeStr=Inherit: Same as first input
  lce/lopt : Gain  Gain=1/loptGLU  SaturateOnIntegerOverflow=on  OutDataTypeStr=Inherit: Same as input  ParamDataTypeStr=Inherit: Same as input
  vmax*lopt : Gain  Gain=vmaxGLU*loptGLU  SaturateOnIntegerOverflow=on  OutDataTypeStr=Inherit: Same as input  ParamDataTypeStr=Inherit: Same as input
  Fmtc : Outport  InitialOutput=0
  Lce : Outport  Port=2  InitialOutput=0
  Vce : Outport  Port=3  InitialOutput=0
  Lse : Outport  Port=4  InitialOutput=0
  A : Outport  Port=5  InitialOutput=0
  wires:
  ECC TransferFcn/1 -> 1/2, A/1
  STIM/1 -> ECC TransferFcn/1
  CE inverse force-velocity relation/1(v[vmax]) -> vmax*lopt/1
  Sum3/1 -> Fv = Fse / (A*Fce)/2
  BE force-length relation/1(fbe [Fmax]) -> Sum4/2
  1/1 -> Sum3/2
  PE force-length relation/1(fpe [Fmax]) -> Sum3/1
  Sum4/1 -> Fv = Fse / (A*Fce)/1
  CE force-length relation/1(fce [Fmax]) -> 1/1
  Constant/1 -> Sum2/1
  Sum2/1 -> Integrator/2
  SE force-length relation/1(fse [Fmax]) -> Sum4/1, Fmax/1
  1/lslack/1 -> SE force-length relation/1(lse [lslack])
  Fmax/1 -> Fmtc/1  "Fmtc"
  lmtc [m]/1 -> Sum/1, Sum2/2  "lmtc"
  vmax*lopt/1 -> Vce/1, Integrator/1  "vce"
  Fv = Fse / (A*Fce)/1 -> CE inverse force-velocity relation/1(Fv[Fmax])  "fv"
  lce/lopt/1 -> PE force-length relation/1(lce [lopt]), BE force-length relation/1(lce [lopt]), CE force-length relation/1(lce [lopt])
  Sum/1 -> Lse/1, 1/lslack/1  "lse"
  Integrator/1 -> Lce/1, lce/lopt/1, Sum/2  "lce"

== system nmc/NMC Muscles/GLU Muscle/GLU Actuation/GLU Link ==
  note: GLUTEUS Attachment
  phi34 [rad] : Inport
  Constant : Constant  Value=lslackGLU+loptGLU
  Constant1 : Constant  Value=rGLU
  Constant2 : Constant  Value=phirefGLU
  Gain2 : Gain  Gain=rhoGLU
  Product : Product  RndMeth=Zero
  Sum2 : Sum  Inputs=|+-
  Sum5 : Sum  Inputs=|+-
  lmtu [m] : Outport
  lever [m] : Outport  Port=2
  wires:
  Gain2/1 -> Sum5/2
  Constant1/1 -> lever [m]/1, Product/2
  Sum2/1 -> Product/1
  Constant2/1 -> Sum2/2
  phi34 [rad]/1 -> Sum2/1
  Product/1 -> Gain2/1
  Sum5/1 -> lmtu [m]/1
  Constant/1 -> Sum5/1

== system nmc/NMC Muscles/GLU Muscle/GLU Control/ Swing Phase ==
  note: GLU Control
  note: Swing Phase Control
  FmGLU : Inport
  Enable : EnablePort  StatesWhenEnabling=reset
  FB Gain2 : Gain  Gain=GainGLU  SaturateOnIntegerOverflow=on  OutDataTypeStr=Inherit: Same as input  ParamDataTypeStr=Inherit: Same as input
  Stimulation Bias3 : Constant  Value=PreStimGLU
  Sum4 : Sum  Inputs=|++  SaturateOnIntegerOverflow=on  InputSameDT=on  OutDataTypeStr=Inherit: Same as first input
  StimGLU : Outport  OutputWhenDisabled=reset  InitialOutput=0
  wires:
  Sum4/1 -> StimGLU/1
  Stimulation Bias3/1 -> Sum4/1
  FmGLU/1 -> FB Gain2/1
  FB Gain2/1 -> Sum4/2

== system nmc/NMC Muscles/GLU Muscle/GLU Control/Stance Phase ==
  note: load bearing potential
  note: Stance Phase Control
  note: GLU Control
  Theta : Inport
  dTheta [rad/s] : Inport  Port=2
  CLdxThigh [N] : Inport  Port=3
  OLonCL : Inport  Port=4
  Enable : EnablePort  StatesWhenEnabling=reset
  Divide : Product
  FB Gain10 : Gain  Gain=SpeedGainGG  SaturateOnIntegerOverflow=on  OutDataTypeStr=Inherit: Same as input  ParamDataTypeStr=Inherit: Same as input
  FB Gain11 : Gain  Gain=PosGainGG  SaturateOnIntegerOverflow=on  OutDataTypeStr=Inherit: Same as input  ParamDataTypeStr=Inherit: Same as input
  FB Gain6 : Gain  Gain=1/DeltaThRef  SaturateOnIntegerOverflow=on  OutDataTypeStr=Inherit: Same as input  ParamDataTypeStr=Inherit: Same as input
  Gain1 : Gain  Gain=0.7
  Gain4 : Gain  Gain=K_swing
  Saturation2 : Saturate  UpperLimit=inf  LowerLimit=0  ZeroCross=off
  Saturation3 : Saturate  UpperLimit=1  LowerLimit=0  ZeroCross=off
  Stimulation Bias6 : Constant  Value=Theta0
  Stimulation Bias7 : Constant  Value=PreStimGG
  Sum10 : Sum  Inputs=|++  SaturateOnIntegerOverflow=on  InputSameDT=on  OutDataTypeStr=Inherit: Same as first input
  Sum12 : Sum  SaturateOnIntegerOverflow=on  InputSameDT=on  OutDataTypeStr=Inherit: Same as first input
  Sum8 : Sum  Inputs=+-  SaturateOnIntegerOverflow=on  InputSameDT=on  OutDataTypeStr=Inherit: Same as first input
  Sum9 : Sum  Inputs=|+-  SaturateOnIntegerOverflow=on  InputSameDT=on  OutDataTypeStr=Inherit: Same as first input
  positive half : Saturate  UpperLimit=inf  LowerLimit=0  ZeroCross=off
  StimGLU : Outport  OutputWhenDisabled=reset  InitialOutput=0
  wires:
  OLonCL/1 -> Gain4/1
  Saturation3/1 -> Sum8/1
  Gain4/1 -> Sum8/2
  Sum8/1 -> Gain1/1
  Divide/1 -> Saturation3/1
  FB Gain6/1 -> Divide/2
  Gain1/1 -> StimGLU/1
  CLdxThigh [N]/1 -> Saturation2/1
  Sum10/1 -> Divide/1
  Saturation2/1 -> FB Gain6/1
  Sum12/1 -> positive half/1
  FB Gain10/1 -> Sum12/2
  FB Gain11/1 -> Sum12/1
  Stimulation Bias7/1 -> Sum10/1
  positive half/1 -> Sum10/2
  Sum9/1 -> FB Gain11/1
  Theta/1 -> Sum9/1
  Stimulation Bias6/1 -> Sum9/2
  dTheta [rad/s]/1 -> FB Gain10/1

== system nmc/NMC Muscles/HFL Muscle /HFL Actuation/ HFL ==
  note: Excitation Contraction Coupling
  note: SOLEUS Muscle-Tendon Dynamics
  STIM : Inport
  lmtc [m] : Inport  Port=2
  1 : Product  Inputs=**  SaturateOnIntegerOverflow=on  InputSameDT=on  OutDataTypeStr=Inherit: Same as first input
  1/lslack : Gain  Gain=1/lslackHFL  SaturateOnIntegerOverflow=on  OutDataTypeStr=Inherit: Same as input  ParamDataTypeStr=Inherit: Same as input
  BE force-length relation : Subsystem
  CE force-length relation : Subsystem
  CE inverse force-velocity relation : Subsystem
  Constant : Constant  Value=lslackHFL
  ECC TransferFcn : simulink_extras/Additional Linear/Transfer Fcn (with initial outputs)  N=[1]  D="[tau  1]"  Y0=preA  U0=0
      settings: AttributesFormatString=pre-activation: %<Y0>
  Fmax : Gain  Gain=FmaxHFL  SaturateOnIntegerOverflow=on  OutDataTypeStr=Inherit: Same as input  ParamDataTypeStr=Inherit: Same as input
  Fv = Fse / (A*Fce) : Product  Inputs=*/  SaturateOnIntegerOverflow=on  InputSameDT=on  OutDataTypeStr=Inherit: Same as first input
  Integrator : Integrator  InitialConditionSource=external  LowerSaturationLimit=0.05
  PE force-length relation : Subsystem
  SE force-length relation : Subsystem
  Sum : Sum  Inputs=|+-  SaturateOnIntegerOverflow=on  InputSameDT=on  OutDataTypeStr=Inherit: Same as first input
  Sum2 : Sum  Inputs=|-+  SaturateOnIntegerOverflow=on  InputSameDT=on  OutDataTypeStr=Inherit: Same as first input
  Sum3 : Sum  SaturateOnIntegerOverflow=on  InputSameDT=on  OutDataTypeStr=Inherit: Same as first input
  Sum4 : Sum  SaturateOnIntegerOverflow=on  InputSameDT=on  OutDataTypeStr=Inherit: Same as first input
  lce/lopt : Gain  Gain=1/loptHFL  SaturateOnIntegerOverflow=on  OutDataTypeStr=Inherit: Same as input  ParamDataTypeStr=Inherit: Same as input
  vmax*lopt : Gain  Gain=vmaxHFL*loptHFL  SaturateOnIntegerOverflow=on  OutDataTypeStr=Inherit: Same as input  ParamDataTypeStr=Inherit: Same as input
  Fmtc : Outport  InitialOutput=0
  Lce : Outport  Port=2  InitialOutput=0
  Vce : Outport  Port=3  InitialOutput=0
  Lse : Outport  Port=4  InitialOutput=0
  A : Outport  Port=5  InitialOutput=0
  wires:
  ECC TransferFcn/1 -> 1/2, A/1
  STIM/1 -> ECC TransferFcn/1
  CE inverse force-velocity relation/1(v[vmax]) -> vmax*lopt/1
  Sum3/1 -> Fv = Fse / (A*Fce)/2
  BE force-length relation/1(fbe [Fmax]) -> Sum4/2
  1/1 -> Sum3/2
  PE force-length relation/1(fpe [Fmax]) -> Sum3/1
  Sum4/1 -> Fv = Fse / (A*Fce)/1
  CE force-length relation/1(fce [Fmax]) -> 1/1
  Constant/1 -> Sum2/1
  Sum2/1 -> Integrator/2
  SE force-length relation/1(fse [Fmax]) -> Sum4/1, Fmax/1
  1/lslack/1 -> SE force-length relation/1(lse [lslack])
  Fmax/1 -> Fmtc/1  "Fmtc"
  lmtc [m]/1 -> Sum/1, Sum2/2  "lmtc"
  vmax*lopt/1 -> Vce/1, Integrator/1  "vce"
  Fv = Fse / (A*Fce)/1 -> CE inverse force-velocity relation/1(Fv[Fmax])  "fv"
  lce/lopt/1 -> PE force-length relation/1(lce [lopt]), BE force-length relation/1(lce [lopt]), CE force-length relation/1(lce [lopt])
  Sum/1 -> Lse/1, 1/lslack/1  "lse"
  Integrator/1 -> Lce/1, lce/lopt/1, Sum/2  "lce"

== system nmc/NMC Muscles/HFL Muscle /HFL Actuation/ HFL Link ==
  note: HFL Attachment
  phi34 [rad] : Inport
  Constant : Constant  Value=lslackHFL+loptHFL
  Constant1 : Constant  Value=rHFL
  Constant2 : Constant  Value=phirefHFL
  Gain2 : Gain  Gain=rhoHFL
  Product : Product  RndMeth=Zero
  Sum2 : Sum  Inputs=|+-
  Sum5 : Sum  Inputs=|++
  lmtu [m] : Outport
  lever [m] : Outport  Port=2
  wires:
  Gain2/1 -> Sum5/2
  Constant1/1 -> lever [m]/1, Product/2
  Sum2/1 -> Product/1
  Constant2/1 -> Sum2/2
  phi34 [rad]/1 -> Sum2/1
  Product/1 -> Gain2/1
  Sum5/1 -> lmtu [m]/1
  Constant/1 -> Sum5/1

== system nmc/NMC Muscles/HFL Muscle /HFL Control/Stance Phase ==
  note: Stance Phase Control
  note: cross leg influence
  note: HFL Control
  note: load bearing potential
  Theta : Inport
  dTheta [rad/s] : Inport  Port=2
  CLdxThigh [N] : Inport  Port=3
  OLonCL : Inport  Port=4
  Enable : EnablePort  StatesWhenEnabling=reset
  Divide1 : Product
  FB Gain10 : Gain  Gain=SpeedGainGG  SaturateOnIntegerOverflow=on  OutDataTypeStr=Inherit: Same as input  ParamDataTypeStr=Inherit: Same as input
  FB Gain11 : Gain  Gain=PosGainGG  SaturateOnIntegerOverflow=on  OutDataTypeStr=Inherit: Same as input  ParamDataTypeStr=Inherit: Same as input
  FB Gain6 : Gain  Gain=1/DeltaThRef  SaturateOnIntegerOverflow=on  OutDataTypeStr=Inherit: Same as input  ParamDataTypeStr=Inherit: Same as input
  Gain3 : Gain  Gain=K_swing
  Saturation1 : Saturate  UpperLimit=1  LowerLimit=0  ZeroCross=off
  Saturation2 : Saturate  UpperLimit=inf  LowerLimit=0  ZeroCross=off
  Stimulation Bias6 : Constant  Value=Theta0
  Stimulation Bias7 : Constant  Value=PreStimGG
  Sum11 : Sum  Inputs=-+|  SaturateOnIntegerOverflow=on  InputSameDT=on  OutDataTypeStr=Inherit: Same as first input
  Sum12 : Sum  SaturateOnIntegerOverflow=on  InputSameDT=on  OutDataTypeStr=Inherit: Same as first input
  Sum13 : Sum  SaturateOnIntegerOverflow=on  InputSameDT=on  OutDataTypeStr=Inherit: Same as first input
  Sum9 : Sum  Inputs=|+-  SaturateOnIntegerOverflow=on  InputSameDT=on  OutDataTypeStr=Inherit: Same as first input
  negative half : Saturate  UpperLimit=0  LowerLimit=-inf  ZeroCross=off
  StimHFL : Outport  OutputWhenDisabled=reset  InitialOutput=0
  Delta_Theta : Outport  Port=2  InitialOutput=0
  wires:
  dTheta [rad/s]/1 -> FB Gain10/1
  Stimulation Bias6/1 -> Sum9/2
  Theta/1 -> Sum9/1
  negative half/1 -> Sum11/1
  Sum9/1 -> FB Gain11/1, Delta_Theta/1
  Stimulation Bias7/1 -> Sum11/2
  FB Gain11/1 -> Sum12/1
  FB Gain10/1 -> Sum12/2
  Sum12/1 -> negative half/1
  Sum13/1 -> StimHFL/1
  Saturation1/1 -> Sum13/1
  Saturation2/1 -> FB Gain6/1
  Sum11/1 -> Divide1/2
  CLdxThigh [N]/1 -> Saturation2/1
  Divide1/1 -> Saturation1/1
  Gain3/1 -> Sum13/2
  FB Gain6/1 -> Divide1/1
  OLonCL/1 -> Gain3/1

== system nmc/NMC Muscles/HFL Muscle /HFL Control/Swing Phase ==
  note: Swing Phase Control
  note: HFL Control
  Delta_Theta : Inport
  LceHFL : Inport  Port=2
  Enable : EnablePort  StatesWhenEnabling=reset
  L+: 0.18 F+: 0.9/Fmax : Gain  Gain=GainHFL  SaturateOnIntegerOverflow=on  OutDataTypeStr=Inherit: Same as input  ParamDataTypeStr=Inherit: Same as input
  L+: 2 : Gain  Gain=GainDeltaTheta  SaturateOnIntegerOverflow=on  OutDataTypeStr=Inherit: Same as input  ParamDataTypeStr=Inherit: Same as input
  Sum2 : Sum  SaturateOnIntegerOverflow=on  InputSameDT=on  OutDataTypeStr=Inherit: Same as first input
  Sum6 : Sum  Inputs=|++  SaturateOnIntegerOverflow=on  InputSameDT=on  OutDataTypeStr=Inherit: Same as first input
  d : Constant  Value=PreStimHFL
  StimHFL : Outport  OutputWhenDisabled=reset  InitialOutput=0
  wires:
  LceHFL/1 -> L+: 0.18 F+: 0.9/Fmax/1
  L+: 0.18 F+: 0.9/Fmax/1 -> Sum6/2
  Delta_Theta/1 -> L+: 2/1
  d/1 -> Sum2/1
  Sum2/1 -> Sum6/1
  L+: 2/1 -> Sum2/2
  Sum6/1 -> StimHFL/1
